simulink model "switched"  (R2020a)
settings: Solver=ode45  StartTime=0.0  StopTime=T  FixedStep=dt  RelTol=0.000001
undefined symbols (not defined in the file or in its folder): den1, den2, num1, num2
libraries: simulink x1
settings Model: Creator=kekatos  LastModifiedBy=kekatos
settings SolverCC: MaxConsecutiveMinStep=5  ZeroCrossAlgorithm=Adaptive

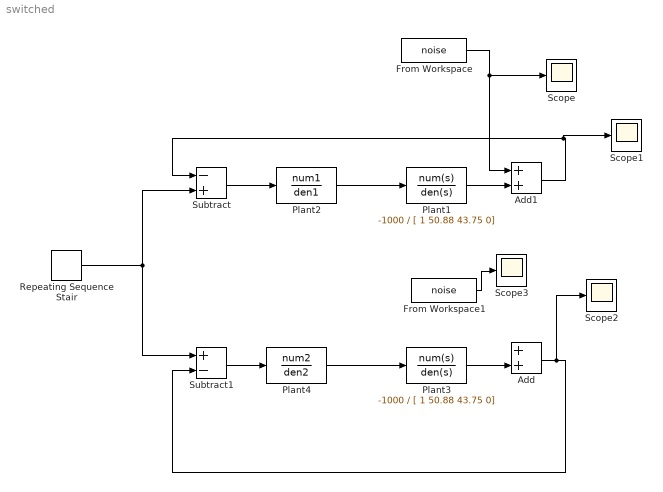
== system switched ==
  Add : Sum
  Add1 : Sum
  From Workspace : FromWorkspace  VariableName=noise
  From Workspace1 : FromWorkspace  VariableName=noise
  Plant1 : TransferFcn  Numerator=-1000  Denominator=[ 1 50.88 43.75 0]
  Plant2 : TransferFcn  Numerator=num1  Denominator=den1
  Plant3 : TransferFcn  Numerator=-1000  Denominator=[ 1 50.88 43.75 0]
  Plant4 : TransferFcn  Numerator=num2  Denominator=den2
  Repeating Sequence Stair : simulink/Sources/Repeating Sequence Stair  OutValues=[1 1 1 1 1 0 0 0 0 0].'  tsamp=2  OutMin=[]  OutMax=[]  OutDataTypeStr=double  OutputDataTypeScalingMode=double  OutDataType=fixdt(0,8)  ConRadixGroup=Best Precision: Vector-wise  OutScaling=2^-12
  Scope{,1..3} (4 alike) : Scope
  Subtract : Sum  Inputs=-+
  Subtract1 : Sum  Inputs=+-
  wires:
  Plant3/1 -> Add/2
  Repeating Sequence Stair/1 -> Subtract/2, Subtract1/1
  Add/1 -> Scope2/1, Subtract1/2
  Plant1/1 -> Add1/2
  Plant4/1 -> Plant3/1
  Subtract1/1 -> Plant4/1
  Subtract/1 -> Plant2/1
  Plant2/1 -> Plant1/1
  From Workspace/1 -> Scope/1, Add1/1
  Add1/1 -> Scope1/1, Subtract/1
  From Workspace1/1 -> Scope3/1
